simulink model "bms"  (R2025b)
settings: Solver=VariableStepAuto  StartTime=0.0  StopTime=3600  RelTol=1e-3
libraries: simulink x2, SignalEditorBlockLib x1

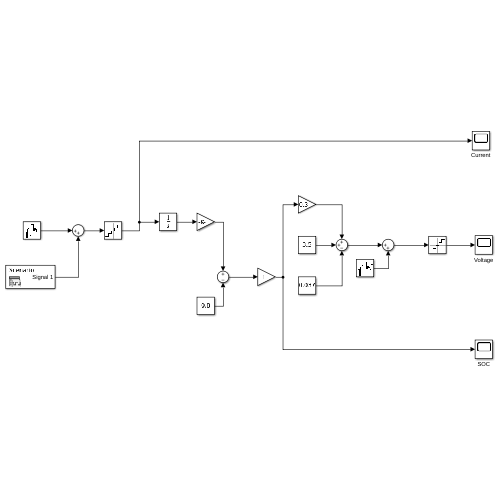
[thumbnail: Simulink's stored preview of the top-level diagram]
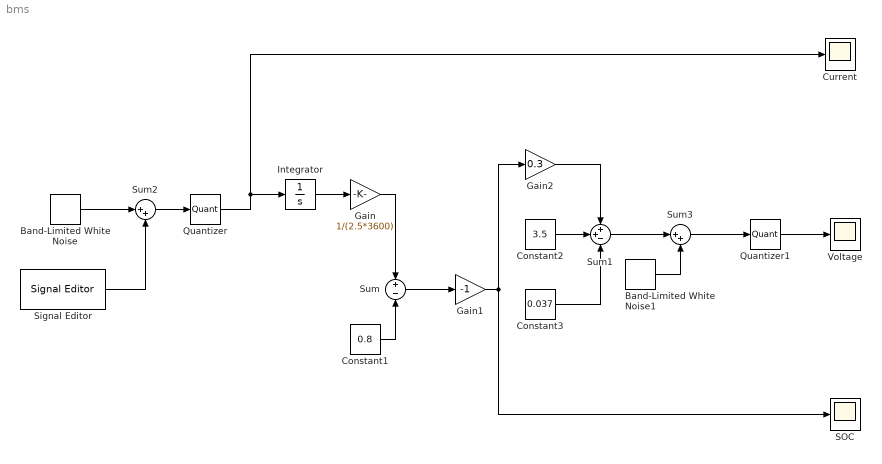
== system bms ==
  Band-Limited White Noise : simulink/Sources/Band-Limited White Noise  Cov=0.001  Ts=1  seed=[23341]
  Band-Limited White Noise1 : simulink/Sources/Band-Limited White Noise  Cov=0.0001  Ts=1  seed=[23342]
  Constant1 : Constant  Value=0.8
  Constant2 : Constant  Value=3.5
  Constant3 : Constant  Value=0.037
  Current : Scope
      settings: ActiveDisplayYMinimum=-0.4325  ActiveDisplayYMaximum=1.0425
  Gain : Gain  Gain=1/(2.5*3600)
  Gain1 : Gain  Gain=-1
  Gain2 : Gain  Gain=0.3
  Integrator : Integrator
  Quantizer : Quantizer  QuantizationInterval=0.001
  Quantizer1 : Quantizer  QuantizationInterval=0.001
  SOC : Scope
      settings: ActiveDisplayYMinimum=0.656795125  ActiveDisplayYMaximum=0.81591165277777777
  Signal Editor : SignalEditorBlockLib/Signal Editor  FileName=Dynamic_Load_Profile.mat  ActiveScenario=Scenario  ActiveSignal=Signal 1  IsBus=off  OutputBusObjectStr=Bus: BusObject  SampleTime=1  ZeroCross=off  OutputAfterFinalValue=Setting to zero  Unit=inherit  PreserveSignalName=on  ApplySigPropsToAllScenarios=on  ApplySigPropsToAllSignals=off  SignalPropertySource=Dialog parameters
  Sum : Sum  Inputs=+-
  Sum1 : Sum  Inputs=++-
  Sum2 : Sum  Inputs=|++
  Sum3 : Sum  Inputs=|++
  Voltage : Scope
      settings: ActiveDisplayYMinimum=3.6266250000000007  ActiveDisplayYMaximum=3.7503750000000005  DataLoggingVariableName=ScopeData2
  wires:
  Integrator/1 -> Gain/1
  Gain/1 -> Sum/1
  Constant1/1 -> Sum/2
  Sum/1 -> Gain1/1
  Gain1/1 -> Gain2/1, SOC/1
  Gain2/1 -> Sum1/1
  Constant2/1 -> Sum1/2
  Constant3/1 -> Sum1/3
  Signal Editor/1 -> Sum2/2
  Band-Limited White Noise/1 -> Sum2/1
  Sum2/1 -> Quantizer/1
  Quantizer/1 -> Current/1, Integrator/1
  Band-Limited White Noise1/1 -> Sum3/2
  Sum1/1 -> Sum3/1
  Sum3/1 -> Quantizer1/1
  Quantizer1/1 -> Voltage/1
